simulink model "sim_3_twolink_task_control_ideal"  (R2021a)
settings: Solver=ode15s  StartTime=0.0  StopTime=20  RelTol=1e-5  EnableMultiTasking=on
values from neighbouring files (symbols this model uses):
  b1 = 0.01    [sim_params.m]    (also in sim_params_force.m)
  b2 = 0.01    [sim_params.m]    (also in sim_params_force.m)
  D = [zeros(n); eye(n)]    [control_comparison_script.m]    (also in gen_twolink_ss.m = reshape([0.0,0.0,0.0,0.0,0.0,0.0,0.0,0.0],[4,2]))
  D_T_Q = D'*Q    [control_comparison_script.m]
  epsilon = 0.1    [control_comparison_script.m]
  g = 9.80665    [sim_params.m]    (also in sim_params_force.m)
  Kpp = place(A,B,p)    [control_comparison_script.m]
  L1x = 0.3    [sim_params.m]    (also in sim_params_force.m)
  L1y = 0.050    (= 0.05)    [sim_params.m]    (also in sim_params_force.m)
  L1z = 0.05    [sim_params.m]    (also in sim_params_force.m)
  L2x = 0.15    [sim_params.m]    (also in sim_params_force.m = 0.3)
  L2y = 0.05    [sim_params.m]    (also in sim_params_force.m)
  L2z = 0.05    [sim_params.m]    (also in sim_params_force.m)
  m1 = m1*1.25    [control_comparison_script.m]    (also in sim_params.m = 2.775; sim_params_force.m = 2.775)
  m2 = m2*1.25    [control_comparison_script.m]    (also in sim_params.m = 1.3875; sim_params_force.m = 2.775)
  param_dev = 15    [control_comparison_script.m]
  rho = [1;1]    [control_comparison_script.m]
  theta1_0 = 0    [sim_params.m]    (also in sim_params_force.m = 1.57079632679)
  theta1_dot_0 = 0    [sim_params.m]    (also in sim_params_force.m)
  theta2_0 = 0    [sim_params.m]    (also in sim_params_force.m = -1.57079632679)
  theta2_dot_0 = 0    [sim_params.m]    (also in sim_params_force.m)
undefined symbols (not defined in the file or in its folder): Kd, Kd_grav, Kd_inv, Ki, Kp, Kp_grav, Kp_inv, N, sigbuilder_block, X, Y, Z
libraries: pid_lib x12, sm_lib x11, nesl_utility x10, spsFirstOrderFilterLib x4, dspmtrx3 x1, simulink x1
(part 3 of 3)

== matlab function sim_3_twolink_task_control_ideal/Controller/PD-gravity Control /Gravity compensation ==
  data: L_1x input; G output; L_2x input; g input; m1 input; m2 input; q1 input; q2 input
function G = G_compensation(L_1x,L_2x,g,m1,m2,q1,q2)
%#codegen

%    This function was generated by the Symbolic Math Toolbox version 8.7.
%    01-Jun-2022 14:38:05

G = [(g.*(L_2x.*m2.*cos(q1+q2)+L_1x.*m1.*cos(q1)+L_1x.*m2.*cos(q1).*2.0))./2.0;(L_2x.*g.*m2.*cos(q1+q2))./2.0];

== matlab function sim_3_twolink_task_control_ideal/Controller/Robust control /MATLAB Function ==
  data: z input; w output; epsilon input; rho input
function w = fcn(z, epsilon, rho)
    z_norm = norm(z);
    if z_norm>=epsilon
        w = (rho/z_norm).*z;
    else
        w = (rho/epsilon).*z;
    end

== matlab function sim_3_twolink_task_control_ideal/THE_XE_YE ==
  data: L_1 input; XE output; L_2 input; theta_1 input; theta_2 input; YE output
function [XE,YE] = THE_XEYE(L_1,L_2,theta_1,theta_2)
%#codegen

%    This function was generated by the Symbolic Math Toolbox version 7.0.
%    05-Sep-2016 11:23:53

XE = L_2.*cos(theta_1+theta_2)+L_1.*cos(theta_1);
if nargout > 1
    YE = L_2.*sin(theta_1+theta_2)+L_1.*sin(theta_1);
end

== matlab function sim_3_twolink_task_control_ideal/Controller/Pole Placement+D Control/disturbance_terms ==
  data: L_1x input; d output; L_2x input; g input; m1 input; m2 input; q1 input; q2 input; q1_D input; q2_D input; q1_DD input; q2_DD input
function d = disturbance_terms(L_1x,L_2x,g,m1,m2,q1,q2,q1_D,q2_D,q1_DD,q2_DD)
%#codegen

%    This function was generated by the Symbolic Math Toolbox version 8.7.
%    10-Jun-2022 15:47:18

d = [(g.*(L_2x.*m2.*cos(q1+q2)+L_1x.*m1.*cos(q1)+L_1x.*m2.*cos(q1).*2.0))./2.0+(L_2x.*m2.*q2_DD.*(L_2x+L_1x.*cos(q2).*2.0))./4.0-(L_1x.*L_2x.*m2.*q2_D.^2.*sin(q2))./2.0+L_1x.*L_2x.*m2.*q1_DD.*cos(q2)-L_1x.*L_2x.*m2.*q1_D.*q2_D.*sin(q2);(L_2x.*g.*m2.*cos(q1+q2))./2.0+(L_2x.*m2.*q1_DD.*(L_2x+L_1x.*cos(q2).*2.0))./4.0+(L_1x.*L_2x.*m2.*q1_D.^2.*sin(q2))./2.0];

== matlab function sim_3_twolink_task_control_ideal/Robot/SIMULINK_MODEL/THE_TH_DD ==
  data: L_1x input; theta_DD output; L_1y input; L_2x input; L_2y input; b1 input; b2 input; g input; m1 input; m2 input; q1 input; q2 input; q1_D input; q2_D input; tau1 input; tau2 input
function theta_DD = THE_TH_DD(L_1x,L_1y,L_2x,L_2y,b1,b2,g,m1,m2,q1,q2,q1_D,q2_D,tau1,tau2)
%#codegen

%    This function was generated by the Symbolic Math Toolbox version 8.7.
%    30-May-2022 13:59:37

et1 = (L_1x.^2.*m1.*4.0+L_1x.^2.*m2.*1.2e+1+L_1y.^2.*m1+L_2x.^2.*m2.*3.0+L_1x.*L_2x.*m2.*cos(q2).*1.2e+1).*(-tau2+b2.*q2_D+(L_1x.*L_2x.*m2.*q1_D.^2.*sin(q2))./2.0+(L_2x.*g.*m2.*cos(q1).*cos(q2))./2.0-(L_2x.*g.*m2.*sin(q1).*sin(q2))./2.0);
et2 = -1.2e+1./(L_2x.^4.*m2.^2.*3.0+L_1x.^2.*L_2x.^2.*m2.^2.*4.8e+1+L_1x.^2.*L_2y.^2.*m2.^2.*1.2e+1+L_2x.^2.*L_2y.^2.*m2.^2.*3.0+L_1x.^2.*L_2x.^2.*m1.*m2.*1.6e+1+L_1x.^2.*L_2y.^2.*m1.*m2.*4.0+L_1y.^2.*L_2x.^2.*m1.*m2.*4.0+L_1y.^2.*L_2y.^2.*m1.*m2-L_1x.^2.*L_2x.^2.*m2.^2.*cos(q2).^2.*3.6e+1+L_1x.*L_2x.^3.*m2.^2.*cos(q2).*1.2e+1+L_1x.*L_2x.*L_2y.^2.*m2.^2.*cos(q2).*1.2e+1);
et3 = ((L_2x.^2+L_1x.*L_2x.*cos(q2).*2.0).*(-tau2+b2.*q2_D+(L_1x.*L_2x.*m2.*q1_D.^2.*sin(q2))./2.0+(L_2x.*g.*m2.*cos(q1).*cos(q2))./2.0-(L_2x.*g.*m2.*sin(q1).*sin(q2))./2.0).*3.6e+1)./(L_2x.^4.*m2.*3.0+L_1x.^2.*L_2x.^2.*m1.*1.6e+1+L_1x.^2.*L_2x.^2.*m2.*4.8e+1+L_1x.^2.*L_2y.^2.*m1.*4.0+L_1y.^2.*L_2x.^2.*m1.*4.0+L_1x.^2.*L_2y.^2.*m2.*1.2e+1+L_1y.^2.*L_2y.^2.*m1+L_2x.^2.*L_2y.^2.*m2.*3.0-L_1x.^2.*L_2x.^2.*m2.*cos(q2).^2.*3.6e+1+L_1x.*L_2x.^3.*m2.*cos(q2).*1.2e+1+L_1x.*L_2x.*L_2y.^2.*m2.*cos(q2).*1.2e+1);
et4 = ((L_2x.^2.*4.0+L_2y.^2).*(tau1-b1.*q1_D-(L_1x.*g.*m1.*cos(q1))./2.0-L_1x.*g.*m2.*cos(q1)+(L_1x.*L_2x.*m2.*q2_D.^2.*sin(q2))./2.0-(L_2x.*g.*m2.*cos(q1).*cos(q2))./2.0+(L_2x.*g.*m2.*sin(q1).*sin(q2))./2.0+L_1x.*L_2x.*m2.*q1_D.*q2_D.*sin(q2)).*1.2e+1)./(L_2x.^4.*m2.*3.0+L_1x.^2.*L_2x.^2.*m1.*1.6e+1+L_1x.^2.*L_2x.^2.*m2.*4.8e+1+L_1x.^2.*L_2y.^2.*m1.*4.0+L_1y.^2.*L_2x.^2.*m1.*4.0+L_1x.^2.*L_2y.^2.*m2.*1.2e+1+L_1y.^2.*L_2y.^2.*m1+L_2x.^2.*L_2y.^2.*m2.*3.0-L_1x.^2.*L_2x.^2.*m2.*cos(q2).^2.*3.6e+1+L_1x.*L_2x.^3.*m2.*cos(q2).*1.2e+1+L_1x.*L_2x.*L_2y.^2.*m2.*cos(q2).*1.2e+1);
theta_DD = [et3+et4;et1.*et2-((L_2x.^2+L_1x.*L_2x.*cos(q2).*2.0).*(tau1-b1.*q1_D-(L_1x.*g.*m1.*cos(q1))./2.0-L_1x.*g.*m2.*cos(q1)+(L_1x.*L_2x.*m2.*q2_D.^2.*sin(q2))./2.0-(L_2x.*g.*m2.*cos(q1).*cos(q2))./2.0+(L_2x.*g.*m2.*sin(q1).*sin(q2))./2.0+L_1x.*L_2x.*m2.*q1_D.*q2_D.*sin(q2)).*3.6e+1)./(L_2x.^4.*m2.*3.0+L_1x.^2.*L_2x.^2.*m1.*1.6e+1+L_1x.^2.*L_2x.^2.*m2.*4.8e+1+L_1x.^2.*L_2y.^2.*m1.*4.0+L_1y.^2.*L_2x.^2.*m1.*4.0+L_1x.^2.*L_2y.^2.*m2.*1.2e+1+L_1y.^2.*L_2y.^2.*m1+L_2x.^2.*L_2y.^2.*m2.*3.0-L_1x.^2.*L_2x.^2.*m2.*cos(q2).^2.*3.6e+1+L_1x.*L_2x.^3.*m2.*cos(q2).*1.2e+1+L_1x.*L_2x.*L_2y.^2.*m2.*cos(q2).*1.2e+1)];

== matlab function sim_3_twolink_task_control_ideal/Robot/SIMULINK_MODEL/MCKGQ ==
  data: L_1x input; M output; L_1y input; L_2x input; L_2y input; b1 input; b2 input; g input; m1 input; m2 input; q1 input; q2 input; q1_D input; q2_D input; tau1 input; tau2 input; C output; K output; G output; Q output
function [M,C,K,G,Q] = MCKGQ(L_1x,L_1y,L_2x,L_2y,b1,b2,g,m1,m2,q1,q2,q1_D,q2_D,tau1,tau2)
%#codegen

%    This function was generated by the Symbolic Math Toolbox version 8.7.
%    30-May-2022 13:59:37

M = reshape([(L_1x.^2.*m1)./3.0+L_1x.^2.*m2+(L_1y.^2.*m1)./1.2e+1+(L_2x.^2.*m2)./4.0+L_1x.*L_2x.*m2.*cos(q2),(L_2x.*m2.*(L_2x+L_1x.*cos(q2).*2.0))./4.0,(L_2x.*m2.*(L_2x+L_1x.*cos(q2).*2.0))./4.0,(m2.*(L_2x.^2.*4.0+L_2y.^2))./1.2e+1],[2,2]);
if nargout > 1
    C = reshape([-L_1x.*L_2x.*m2.*q2_D.*sin(q2),(L_1x.*L_2x.*m2.*q1_D.*sin(q2))./2.0,L_1x.*L_2x.*m2.*q2_D.*sin(q2).*(-1.0./2.0),0.0],[2,2]);
end
if nargout > 2
    K = reshape([0.0,0.0,0.0,0.0],[2,2]);
end
if nargout > 3
    G = [(g.*(L_2x.*m2.*cos(q1+q2)+L_1x.*m1.*cos(q1)+L_1x.*m2.*cos(q1).*2.0))./2.0;(L_2x.*g.*m2.*cos(q1+q2))./2.0];
end
if nargout > 4
    Q = [tau1-b1.*q1_D;tau2-b2.*q2_D];
end

== matlab function sim_3_twolink_task_control_ideal/Robot/SIMULINK_MODEL/MATLAB Function1 ==
  data: M input; the_cond output
function the_cond = COND(M)
%#codegen

the_cond = cond(M);

end

== matlab function sim_3_twolink_task_control_ideal/Controller/PD-feedforward-gravity Control/Gravity compensation ==
  data: L_1x input; G output; L_2x input; g input; m1 input; m2 input; q1 input; q2 input
function G = G_compensation(L_1x,L_2x,g,m1,m2,q1,q2)
%#codegen

%    This function was generated by the Symbolic Math Toolbox version 8.7.
%    01-Jun-2022 14:38:05

G = [(g.*(L_2x.*m2.*cos(q1+q2)+L_1x.*m1.*cos(q1)+L_1x.*m2.*cos(q1).*2.0))./2.0;(L_2x.*g.*m2.*cos(q1+q2))./2.0];

== matlab function sim_3_twolink_task_control_ideal/Controller/Inverse Dynamics control /MCKGQ ==
  data: L_1x input; M output; L_1y input; L_2x input; L_2y input; b1 input; b2 input; g input; m1 input; m2 input; q1 input; q2 input; q1_D input; q2_D input; tau1 input; tau2 input; C output; K output; G output; Q output
function [M,C,K,G,Q] = MCKGQ(L_1x,L_1y,L_2x,L_2y,b1,b2,g,m1,m2,q1,q2,q1_D,q2_D,tau1,tau2)
%#codegen

%    This function was generated by the Symbolic Math Toolbox version 8.7.
%    30-May-2022 13:59:37

M = reshape([(L_1x.^2.*m1)./3.0+L_1x.^2.*m2+(L_1y.^2.*m1)./1.2e+1+(L_2x.^2.*m2)./4.0+L_1x.*L_2x.*m2.*cos(q2),(L_2x.*m2.*(L_2x+L_1x.*cos(q2).*2.0))./4.0,(L_2x.*m2.*(L_2x+L_1x.*cos(q2).*2.0))./4.0,(m2.*(L_2x.^2.*4.0+L_2y.^2))./1.2e+1],[2,2]);
if nargout > 1
    C = reshape([-L_1x.*L_2x.*m2.*q2_D.*sin(q2),(L_1x.*L_2x.*m2.*q1_D.*sin(q2))./2.0,L_1x.*L_2x.*m2.*q2_D.*sin(q2).*(-1.0./2.0),0.0],[2,2]);
end
if nargout > 2
    K = reshape([0.0,0.0,0.0,0.0],[2,2]);
end
if nargout > 3
    G = [(g.*(L_2x.*m2.*cos(q1+q2)+L_1x.*m1.*cos(q1)+L_1x.*m2.*cos(q1).*2.0))./2.0;(L_2x.*g.*m2.*cos(q1+q2))./2.0];
end
if nargout > 4
    Q = [tau1-b1.*q1_D;tau2-b2.*q2_D];
end
